simulink model "TEModel_random"  (Simulink 8.3)
settings: Solver=ode1  SolverMode=SingleTasking  StartTime=0.0  StopTime=72  FixedStep=Ts_base  MaxStep=Ts_base  MinStep=1e-6  RelTol=1e-6
PreLoadFcn:
  | initModel
StopFcn:
  | TEplot
undefined symbols (not defined in the file): Ts_base, Ts_save
libraries: VAlib x28, TElib x18
(part 1 of 9)
settings Model: Creator=pydipalli  LastModifiedBy=lexx
settings DataIOCC: LimitDataPoints=off  LoadInitialState=on  SaveFinalState=on  SaveFormat=Structure  SaveOutput=off  SaveTime=off  SignalLoggingName=sigsOut
settings OptimizationCC: ExpressionDepthLimit=2147483647  InitFltsAndDblsToZero=on
settings DebuggingCC: SaveWithDisabledLinksMsg=none  SaveWithParameterizedLinksMsg=none  SignalResolutionControl=TryResolveAllWithWarning  SolverPrmCheckMsg=none  MultiTaskDSMMsg=warning  MultiTaskCondExecSysMsg=none  FcnCallInpInsideContextMsg=UseLocalSettings
settings HardwareCC: TargetUnknown=on
settings RTWCC: IncludeERTFirstTime=on
settings GRTTargetCC: TargetFcnLib=ansi_tfl_tmw.mat

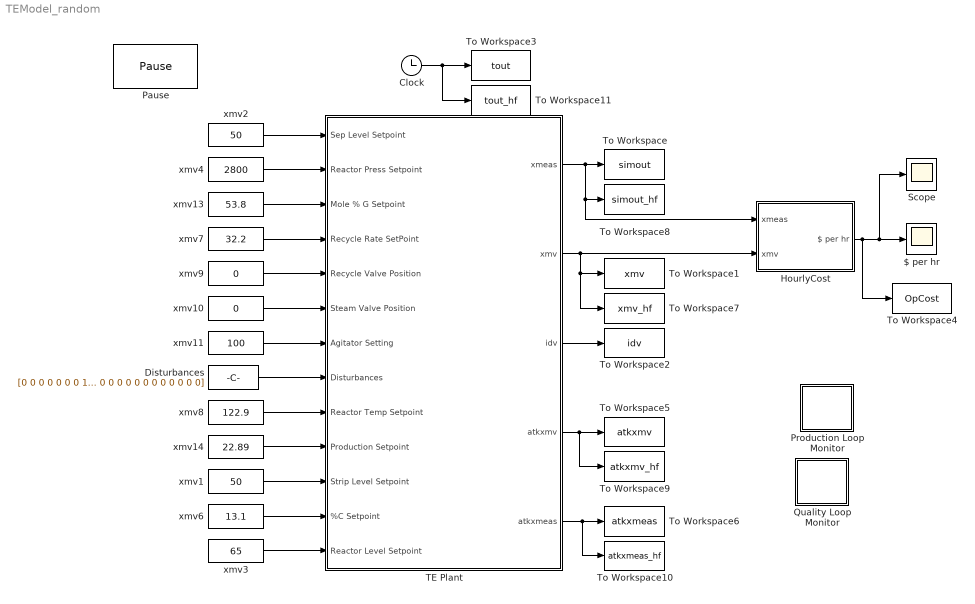
== system TEModel_random ==
  $ per hr : Scope
      settings: YMin=25  YMax=225  SaveName=OpCost  SampleInput=on  SampleTime=Ts_save
  Clock : Clock
  Disturbances : Constant  Value=[0 0 0 0 0 0 0 1 0 0 0 0 0 0 0 0 0 0 0 0]
  HourlyCost : Subsystem
  Pause : TElib/Pause  Value=-1
  Production Loop Monitor : Subsystem
  Quality Loop Monitor : Subsystem
  Scope : Scope
      settings: YMin=75  YMax=325  SaveName=ScopeData19
  TE Plant : Subsystem
  To Workspace : ToWorkspace  VariableName=simout  SampleTime=Ts_save
  To Workspace1 : ToWorkspace  VariableName=xmv  SampleTime=Ts_save
  To Workspace10 : ToWorkspace  VariableName=atkxmeas_hf  SampleTime=-1
  To Workspace11 : ToWorkspace  VariableName=tout_hf  SampleTime=-1
  To Workspace2 : ToWorkspace  VariableName=idv  SampleTime=Ts_save
  To Workspace3 : ToWorkspace  VariableName=tout  SampleTime=Ts_save
  To Workspace4 : ToWorkspace  VariableName=OpCost  SampleTime=Ts_save
  To Workspace5 : ToWorkspace  VariableName=atkxmv  SampleTime=Ts_save
  To Workspace6 : ToWorkspace  VariableName=atkxmeas  SampleTime=Ts_save
  To Workspace7 : ToWorkspace  VariableName=xmv_hf  SampleTime=-1
  To Workspace8 : ToWorkspace  VariableName=simout_hf  SampleTime=-1
  To Workspace9 : ToWorkspace  VariableName=atkxmv_hf  SampleTime=-1
  xmv1 : Constant  Value=50
  xmv10 : Constant  Value=0
  xmv11 : Constant  Value=100
  xmv13 : Constant  Value=53.8
  xmv14 : Constant  Value=22.89
  xmv2 : Constant  Value=50
  xmv3 : Constant  Value=65
  xmv4 : Constant  Value=2800
  xmv6 : Constant  Value=13.1
  xmv7 : Constant  Value=32.2
  xmv8 : Constant  Value=122.9
  xmv9 : Constant  Value=0
  wires:
  TE Plant/1(xmeas) -> To Workspace8/1, HourlyCost/1(xmeas), To Workspace/1
  xmv1/1 -> TE Plant/11(Strip Level Setpoint)
  xmv2/1 -> TE Plant/1(Sep Level Setpoint)
  xmv3/1 -> TE Plant/13(Reactor Level Setpoint)
  xmv4/1 -> TE Plant/2(Reactor Press Setpoint)
  xmv8/1 -> TE Plant/9(Reactor Temp Setpoint)
  xmv6/1 -> TE Plant/12(%C Setpoint)
  xmv7/1 -> TE Plant/4(Recycle Rate SetPoint)
  TE Plant/2(xmv) -> To Workspace7/1, To Workspace1/1, HourlyCost/2(xmv)
  TE Plant/3(idv) -> To Workspace2/1
  Clock/1 -> To Workspace11/1, To Workspace3/1
  HourlyCost/1($ per hr) -> Scope/1, $ per hr/1, To Workspace4/1
  xmv9/1 -> TE Plant/5(Recycle Valve Position)
  xmv10/1 -> TE Plant/6(Steam Valve Position)
  xmv11/1 -> TE Plant/7(Agitator Setting)
  Disturbances/1 -> TE Plant/8(Disturbances)
  xmv13/1 -> TE Plant/3(Mole % G Setpoint)
  xmv14/1 -> TE Plant/10(Production Setpoint)
  TE Plant/4(atkxmv) -> To Workspace9/1, To Workspace5/1
  TE Plant/5(atkxmeas) -> To Workspace10/1, To Workspace6/1

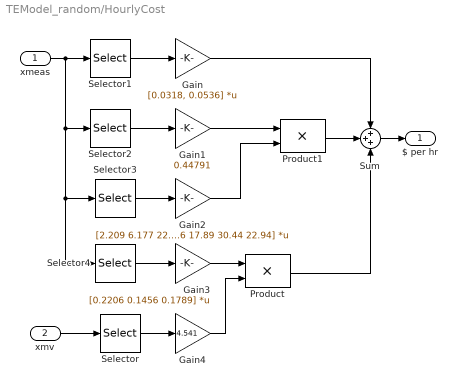
== system TEModel_random/HourlyCost ==
  xmeas : Inport  PortDimensions=41
  xmv : Inport  Port=2  PortDimensions=12
  Gain : Gain  Gain=[0.0318, 0.0536]  Multiplication=Matrix(K*u)  SaturateOnIntegerOverflow=on  OutDataTypeStr=Inherit: Same as input  ParamDataTypeStr=Inherit: Same as input
  Gain1 : Gain  Gain=0.44791  SaturateOnIntegerOverflow=on  OutDataTypeStr=Inherit: Same as input  ParamDataTypeStr=Inherit: Same as input
  Gain2 : Gain  Gain=[2.209 6.177 22.06 14.56 17.89 30.44 22.94]  Multiplication=Matrix(K*u)  SaturateOnIntegerOverflow=on  OutDataTypeStr=Inherit: Same as input  ParamDataTypeStr=Inherit: Same as input
  Gain3 : Gain  Gain=[0.2206 0.1456 0.1789]  Multiplication=Matrix(K*u)  SaturateOnIntegerOverflow=on  OutDataTypeStr=Inherit: Same as input  ParamDataTypeStr=Inherit: Same as input
  Gain4 : Gain  Gain=4.541  SaturateOnIntegerOverflow=on  OutDataTypeStr=Inherit: Same as input  ParamDataTypeStr=Inherit: Same as input
  Product : Product  SaturateOnIntegerOverflow=on  OutDataTypeStr=Inherit: Same as first input
  Product1 : Product  SaturateOnIntegerOverflow=on  OutDataTypeStr=Inherit: Same as first input
  Selector : Selector  InputPortWidth=12  Indices=8
  Selector1 : Selector  InputPortWidth=41  Indices=[19 20]
  Selector2 : Selector  InputPortWidth=41  Indices=[10]
  Selector3 : Selector  InputPortWidth=41  Indices=[29, 31:36]
  Selector4 : Selector  InputPortWidth=41  Indices=[37:39]
  Sum : Sum  Inputs=+++  SaturateOnIntegerOverflow=on
  $ per hr : Outport
  wires:
  xmv/1 -> Selector/1
  xmeas/1 -> Selector1/1, Selector2/1, Selector3/1, Selector4/1
  Selector1/1 -> Gain/1
  Selector2/1 -> Gain1/1
  Selector3/1 -> Gain2/1
  Selector4/1 -> Gain3/1
  Selector/1 -> Gain4/1
  Gain3/1 -> Product/1
  Gain4/1 -> Product/2
  Sum/1 -> $ per hr/1
  Product/1 -> Sum/3
  Gain/1 -> Sum/1
  Product1/1 -> Sum/2
  Gain1/1 -> Product1/1
  Gain2/1 -> Product1/2

== system TEModel_random/Production Loop Monitor ==
  Mux2 : Mux  Inputs=2
  Production : Scope
      settings: YMin=20  YMax=28  SaveName=Production  SampleInput=on  SampleTime=Ts_save
  To Workspace4 : ToWorkspace  VariableName=production  SampleTime=Ts_save
  wires:
  Mux2/1 -> To Workspace4/1, Production/1
  [xmeas17] -> Mux2/2
  [Prodsp] -> Mux2/1

== system TEModel_random/Quality Loop Monitor ==
  Mux2 : Mux  Inputs=2
  Quality : Scope
      settings: YMin=51.5  YMax=56  SaveName=Quality  SampleInput=on  SampleTime=Ts_save
  Scope : Scope
      settings: YMin=52.5  YMax=55.25  SaveName=ScopeData10
  wires:
  [PctGsp] -> Mux2/1
  [xmeas40] -> Scope/1, Mux2/2
  Mux2/1 -> Quality/1

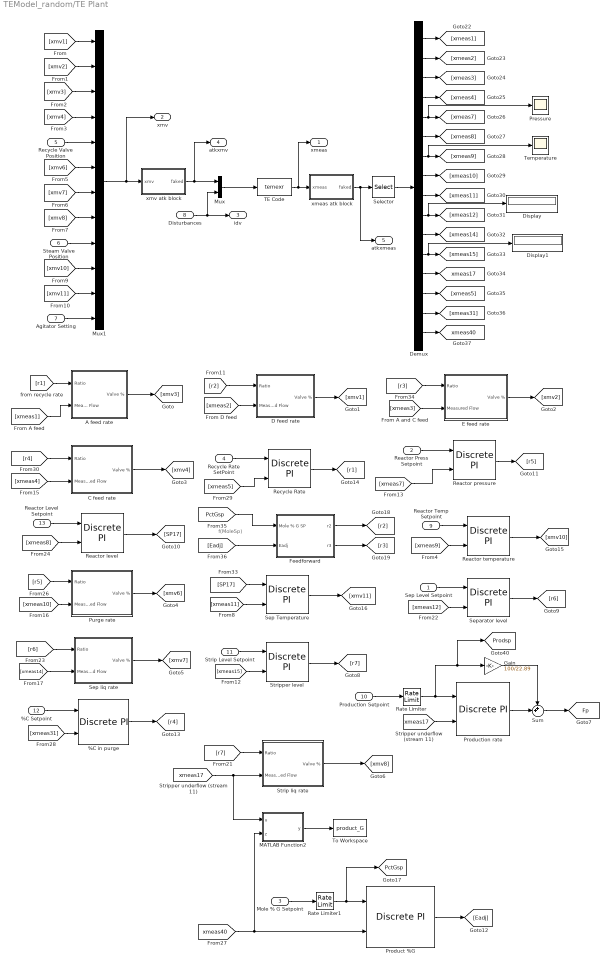
== system TEModel_random/TE Plant ==
  note: f(MoleSp)
  Sep Level Setpoint : Inport
  Reactor Press Setpoint : Inport  Port=2
  Mole % G Setpoint : Inport  Port=3
  Recycle Rate SetPoint : Inport  Port=4
  Recycle Valve Position : Inport  Port=5
  Steam Valve Position : Inport  Port=6
  Agitator Setting : Inport  Port=7
  Disturbances : Inport  Port=8
  Reactor Temp Setpoint : Inport  Port=9
  Production Setpoint : Inport  Port=10
  Strip Level Setpoint : Inport  Port=11
  %C Setpoint : Inport  Port=12
  Reactor Level Setpoint : Inport  Port=13
  %C in purge : TElib/Discrete PI  Kc=0.0009  Ti=562/60  Ts=Ts_base  x0=r4_0  Hi=200  Lo=0
  A feed rate : Subsystem
  C feed rate : Subsystem
  D feed rate : Subsystem
  Demux : Demux  Outputs=16
  Display : Display
  Display1 : Display
  E feed rate : Subsystem
  Feedforward : Subsystem
  Gain : Gain  Gain=100/22.89  SaturateOnIntegerOverflow=on  OutDataTypeStr=Inherit: Same as input  ParamDataTypeStr=Inherit: Same as input
  MATLAB Function2 : MATLAB Function  TreatAsAtomicUnit=on
  Mux : Mux  Inputs=2
  Mux1 : Mux  Inputs=12
  Pressure : Scope
      settings: YMin=2700  YMax=2900  SampleInput=on  SampleTime=Ts_save
  Product %G : TElib/Discrete PI  Kc=-0.032  Ti=100/60  Ts=Ts_base  x0=Eadj_0  Hi=inf  Lo=-inf
  Production rate : TElib/Discrete PI  Kc=3.2  Ti=120/60  Ts=Ts_base  x0=0  Hi=20  Lo=-20
  Purge rate : Subsystem
  Rate Limiter : RateLimiter  RisingSlewLimit=0.3*22.95/24  FallingSlewLimit=-0.3*22.95/24
  Rate Limiter1 : RateLimiter  RisingSlewLimit=50/24  FallingSlewLimit=-50/24
  Reactor level : TElib/Discrete PI  Kc=0.8  Ti=60/60  Ts=Ts_base  x0=SP17_0  Hi=120  Lo=0
  Reactor pressure : TElib/Discrete PI  Kc=-1e-4  Ti=20/60  Ts=Ts_base  x0=r5_0  Hi=100  Lo=0
  Reactor temperature : TElib/Discrete PI  Kc=-8  Ti=7.5/60  Ts=Ts_base  x0=xmv10_0  Hi=100  Lo=0
  Recycle Rate : TElib/Discrete PI  Kc=0.00125  Ti=120/60  Ts=Ts_base  x0=r1_0  Hi=200  Lo=0
  Selector : Selector  InputPortWidth=41  Indices=[1:4, 7:12, 14, 15, 17, 5, 31, 40]
  Sep Temperature : TElib/Discrete PI  Kc=-4  Ti=15/60  Ts=Ts_base  x0=xmv11_0  Hi=100  Lo=0
  Sep liq rate : Subsystem
  Separator level : TElib/Discrete PI  Kc=-1e-3  Ti=200/60  Ts=Ts_base  x0=r6_0  Hi=100  Lo=0
  Strip liq rate : Subsystem
  Stripper level : TElib/Discrete PI  Kc=-2e-4  Ti=200/60  Ts=Ts_base  x0=r7_0  Hi=100  Lo=0
  Sum : Sum  Inputs=++|  SaturateOnIntegerOverflow=on
  TE Code : S-Function  FunctionName=temexr  Parameters=[],[]  EnableBusSupport=off
  Temperature : Scope
      settings: YMin=120  YMax=130  SampleInput=on  SampleTime=Ts_save
  To Workspace : ToWorkspace  VariableName=product_G  SampleTime=-1
  xmeas atk block : Subsystem
  xmv atk block : Subsystem
  xmeas : Outport
  xmv : Outport  Port=2
  idv : Outport  Port=3
  atkxmv : Outport  Port=4
  atkxmeas : Outport  Port=5
  tag scope: Fp=global, PctGsp=global, Prodsp=global, xmeas17=global, xmeas40=global
  wires:
  Mux/1 -> TE Code/1
  Disturbances/1 -> Mux/2, idv/1
  TE Code/1 -> xmeas atk block/1(xmeas), xmeas/1
  [xmv1] -> Mux1/1
  [xmv2] -> Mux1/2
  [xmv3] -> Mux1/3
  [xmv4] -> Mux1/4
  Recycle Valve Position/1 -> Mux1/5
  [xmv6] -> Mux1/6
  [xmv7] -> Mux1/7
  [xmv8] -> Mux1/8
  Steam Valve Position/1 -> Mux1/9
  [xmv10] -> Mux1/10
  [xmv11] -> Mux1/11
  Agitator Setting/1 -> Mux1/12
  A feed rate/1(Valve %) -> [xmv3]
  D feed rate/1(Valve %) -> [xmv1]
  E feed rate/1(Valve %) -> [xmv2]
  Purge rate/1(Valve %) -> [xmv6]
  [xmeas17] -> Strip liq rate/2(Measured Flow), MATLAB Function2/1(u)
  [r7] -> Strip liq rate/1(Ratio)
  Sep Level Setpoint/1 -> Separator level/1
  Separator level/1 -> [r6]
  Reactor Press Setpoint/1 -> Reactor pressure/1
  Reactor pressure/1 -> [r5]
  Product %G/1 -> [Eadj]
  Recycle Rate SetPoint/1 -> Recycle Rate/1
  Recycle Rate/1 -> [r1]
  [r1] -> A feed rate/1(Ratio)
  Sep Temperature/1 -> [xmv11]
  [r2] -> D feed rate/1(Ratio)
  [r3] -> E feed rate/1(Ratio)
  Mux1/1 -> xmv atk block/1(xmv), xmv/1
  Demux/1 -> [xmeas1]
  Demux/2 -> [xmeas2]
  Demux/3 -> [xmeas3]
  Demux/4 -> [xmeas4]
  Demux/5 -> [xmeas7], Pressure/1
  Demux/6 -> [xmeas8]
  Demux/7 -> [xmeas9], Temperature/1
  Demux/8 -> [xmeas10]
  Demux/9 -> [xmeas11]
  Demux/10 -> [xmeas12], Display/1
  Demux/11 -> [xmeas14]
  Demux/12 -> [xmeas15], Display1/1
  Demux/13 -> [xmeas17]
  Demux/14 -> [xmeas5]
  Demux/15 -> [xmeas31]
  Demux/16 -> [xmeas40]
  [r4] -> C feed rate/1(Ratio)
  Rate Limiter1/1 -> Product %G/1, [PctGsp]
  Mole % G Setpoint/1 -> Rate Limiter1/1
  C feed rate/1(Valve %) -> [xmv4]
  [xmeas3] -> E feed rate/2(Measured Flow)
  MATLAB Function2/1(y) -> To Workspace/1
  [r5] -> Purge rate/1(Ratio)
  [SP17] -> Sep Temperature/1
  [xmeas11] -> Sep Temperature/2
  [xmeas1] -> A feed rate/2(Measured Flow)
  [xmeas2] -> D feed rate/2(Measured Flow)
  Reactor Temp Setpoint/1 -> Reactor temperature/1
  Reactor temperature/1 -> [xmv10]
  [xmeas9] -> Reactor temperature/2
  Rate Limiter/1 -> Production rate/1, [Prodsp], Gain/1
  Production Setpoint/1 -> Rate Limiter/1
  Sum/1 -> [Fp]
  Production rate/1 -> Sum/2
  Gain/1 -> Sum/1
  Strip Level Setpoint/1 -> Stripper level/1
  Stripper level/1 -> [r7]
  Sep liq rate/1(Valve %) -> [xmv7]
  [r6] -> Sep liq rate/1(Ratio)
  [xmeas14] -> Sep liq rate/2(Measured Flow)
  %C Setpoint/1 -> %C in purge/1
  %C in purge/1 -> [r4]
  [xmeas31] -> %C in purge/2
  Reactor Level Setpoint/1 -> Reactor level/1
  Reactor level/1 -> [SP17]
  [PctGsp] -> Feedforward/1(Mole % G SP)
  [Eadj] -> Feedforward/2(Eadj)
  Feedforward/1(r2) -> [r2]
  Feedforward/2(r3) -> [r3]
  [xmeas40] -> Product %G/2, MATLAB Function2/2(z)
  [xmeas15] -> Stripper level/2
  [xmeas8] -> Reactor level/2
  [xmeas17] -> Production rate/2
  Strip liq rate/1(Valve %) -> [xmv8]
  [xmeas5] -> Recycle Rate/2
  [xmeas10] -> Purge rate/2(Measured Flow)
  [xmeas4] -> C feed rate/2(Measured Flow)
  [xmeas12] -> Separator level/2
  xmv atk block/1(faked) -> atkxmv/1, Mux/1
  [xmeas7] -> Reactor pressure/2
  xmeas atk block/1(faked) -> atkxmeas/1, Selector/1
  Selector/1 -> Demux/1

== system TEModel_random/TE Plant/A feed rate ==
  Ratio : Inport
  Measured Flow : Inport  Port=2
  Discrete PI : TElib/Discrete PI  Kc=0.01  Ti=0.001/60  Ts=Ts_base  x0=xmv3_0  Hi=100  Lo=0
  Product : Product  SaturateOnIntegerOverflow=on  OutDataTypeStr=Inherit: Same as first input
  Valve % : Outport
  wires:
  Discrete PI/1 -> Valve %/1
  Ratio/1 -> Product/1
  [Fp] -> Product/2
  Measured Flow/1 -> Discrete PI/2
  Product/1 -> Discrete PI/1

== system TEModel_random/TE Plant/C feed rate ==
  Ratio : Inport
  Measured Flow : Inport  Port=2
  Discrete PI : TElib/Discrete PI  Kc=0.003  Ti=0.001/60  Ts=Ts_base  x0=xmv4_0  Hi=100  Lo=0
  Product : Product  SaturateOnIntegerOverflow=on  OutDataTypeStr=Inherit: Same as first input
  Valve % : Outport
  wires:
  Product/1 -> Discrete PI/1
  Measured Flow/1 -> Discrete PI/2
  [Fp] -> Product/2
  Ratio/1 -> Product/1
  Discrete PI/1 -> Valve %/1

== system TEModel_random/TE Plant/D feed rate ==
  Ratio : Inport
  Measured Flow : Inport  Port=2
  Discrete PI : TElib/Discrete PI  Kc=1.6e-6  Ti=0.001/60  Ts=Ts_base  x0=xmv1_0  Hi=100  Lo=0
  Product : Product  SaturateOnIntegerOverflow=on  OutDataTypeStr=Inherit: Same as first input
  Valve % : Outport
  wires:
  Product/1 -> Discrete PI/1
  Measured Flow/1 -> Discrete PI/2
  [Fp] -> Product/2
  Ratio/1 -> Product/1
  Discrete PI/1 -> Valve %/1

== system TEModel_random/TE Plant/E feed rate ==
  Ratio : Inport
  Measured Flow : Inport  Port=2
  Discrete PI : TElib/Discrete PI  Kc=1.8e-6  Ti=0.001/60  Ts=Ts_base  x0=xmv2_0  Hi=100  Lo=0
  Product : Product  SaturateOnIntegerOverflow=on  OutDataTypeStr=Inherit: Same as first input
  Valve % : Outport
  wires:
  Product/1 -> Discrete PI/1
  Measured Flow/1 -> Discrete PI/2
  [Fp] -> Product/2
  Ratio/1 -> Product/1
  Discrete PI/1 -> Valve %/1

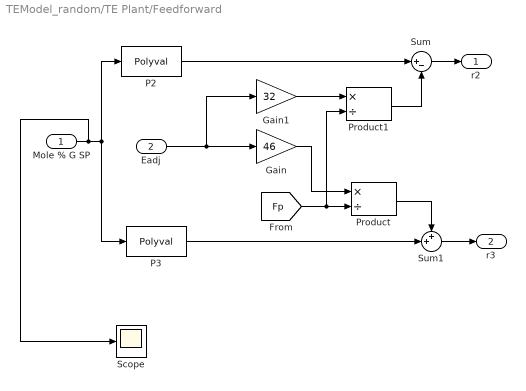
== system TEModel_random/TE Plant/Feedforward ==
  Mole % G SP : Inport
  Eadj : Inport  Port=2
  Gain : Gain  Gain=46  SaturateOnIntegerOverflow=on  OutDataTypeStr=Inherit: Same as input  ParamDataTypeStr=Inherit: Same as input
  Gain1 : Gain  Gain=32  SaturateOnIntegerOverflow=on  OutDataTypeStr=Inherit: Same as input  ParamDataTypeStr=Inherit: Same as input
  P2 : Polyval  Coefs="[1.5192e-003  5.9446e-001  2.7690e-001]"
  P3 : Polyval  Coefs="[-1.1377e-003 -8.0893e-001  9.1060e+001]"
  Product : Product  Inputs=*/  SaturateOnIntegerOverflow=on  OutDataTypeStr=Inherit: Same as first input
  Product1 : Product  Inputs=*/  SaturateOnIntegerOverflow=on  OutDataTypeStr=Inherit: Same as first input
  Scope : Scope
      settings: YMin=53.8  YMax=53.8  SaveName=ScopeData4
  Sum : Sum  Inputs=|+-  SaturateOnIntegerOverflow=on
  Sum1 : Sum  Inputs=++|  SaturateOnIntegerOverflow=on
  r2 : Outport
  r3 : Outport  Port=2
  wires:
  Sum/1 -> r2/1
  P2/1 -> Sum/1
  Sum1/1 -> r3/1
  P3/1 -> Sum1/2
  Product/1 -> Sum1/1
  [Fp] -> Product/2, Product1/2
  Gain/1 -> Product/1
  Eadj/1 -> Gain/1, Gain1/1
  Product1/1 -> Sum/2
  Gain1/1 -> Product1/1
  Mole % G SP/1 -> Scope/1, P2/1, P3/1

== system TEModel_random/TE Plant/Purge rate ==
  Ratio : Inport
  Measured Flow : Inport  Port=2
  Discrete PI : TElib/Discrete PI  Kc=0.01  Ti=0.001/60  Ts=Ts_base  x0=xmv6_0  Hi=100  Lo=0
  Product : Product  SaturateOnIntegerOverflow=on  OutDataTypeStr=Inherit: Same as first input
  Valve % : Outport
  wires:
  Discrete PI/1 -> Valve %/1
  Ratio/1 -> Product/1
  [Fp] -> Product/2
  Measured Flow/1 -> Discrete PI/2
  Product/1 -> Discrete PI/1

== system TEModel_random/TE Plant/Sep liq rate ==
  Ratio : Inport
  Measured Flow : Inport  Port=2
  Discrete PI : TElib/Discrete PI  Kc=4e-4  Ti=0.001/60  Ts=Ts_base  x0=xmv7_0  Hi=100  Lo=0
  Product : Product  SaturateOnIntegerOverflow=on  OutDataTypeStr=Inherit: Same as first input
  Valve % : Outport
  wires:
  Product/1 -> Discrete PI/1
  Measured Flow/1 -> Discrete PI/2
  [Fp] -> Product/2
  Ratio/1 -> Product/1
  Discrete PI/1 -> Valve %/1

== system TEModel_random/TE Plant/Strip liq rate ==
  Ratio : Inport
  Measured Flow : Inport  Port=2
  Discrete PI : TElib/Discrete PI  Kc=4e-4  Ti=0.001/60  Ts=Ts_base  x0=xmv8_0  Hi=100  Lo=0
  Product : Product  SaturateOnIntegerOverflow=on  OutDataTypeStr=Inherit: Same as first input
  Valve % : Outport
  wires:
  Discrete PI/1 -> Valve %/1
  Ratio/1 -> Product/1
  [Fp] -> Product/2
  Measured Flow/1 -> Discrete PI/2
  Product/1 -> Discrete PI/1
